simulink model "foc"  (R2023a)
settings: Solver=VariableStepAuto  StartTime=0.0  StopTime=20  FixedStep=1e-4  MaxStep=1e-4  RelTol=1e-3
values from neighbouring files (symbols this model uses):
  A = exp(F*Ts)    [data.m]
  V = 12    [data.m]
libraries: spsMosfetLib x6, spsPermanentMagnetSynchronousMachineLib x1, spsCurrentMeasurementLib x1, spsDCVoltageSourceLib x1, spsGroundLib x1, slpidlib x1, simulink x1, mcbsensorlessestimatorlib x1, sps_lib x1
settings Model: Creator=Daniil  LastModifiedBy=Daniil

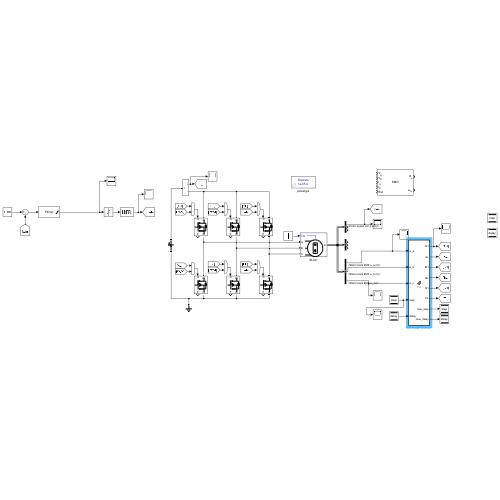
[thumbnail: Simulink's stored preview of the top-level diagram]
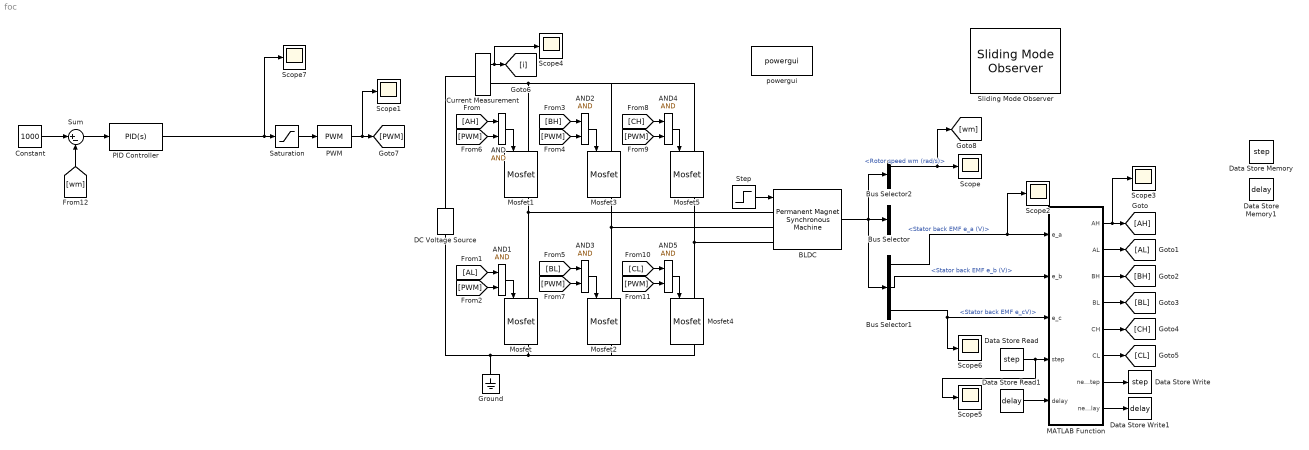
== system foc ==
  AND{,1..5} (6 alike) : Logic  IconShape=distinctive  AllPortsSameDT=off  OutDataTypeStr=boolean
  BLDC : spsPermanentMagnetSynchronousMachineLib/Permanent Magnet Synchronous Machine  NbPhases=3  FluxDistribution=Trapezoidal  RotorType=Round  MechanicalLoad=Torque Tm  PresetModel=No  ShowDetailedParameters=on  MeasurementBus=off  Resistance=0.18  Inductance=0.000835  dqInductances=[8.5e-3,8.5e-3]  La=0.000835  MachineConstant=Flux linkage established by magnets (V.s)  Flux=0.00108515  VoltageCst=0.90909  TorqueCst=0.0086812  Flat=120  Mechanical=[0.0621417 0.000303448 4]  PolePairs=4  InitialConditions=[10,0, 0,0]  InitialConditions5ph=[0 0 0 0 0 0]  RefAngle=90 degrees behind phase A axis (modified Park)  IterativeDiscreteModel=Trapezoidal non iterative  TsBlock=-1  TsPowergui=0
  Bus Selector : BusSelector  OutputSignals=Stator current is_a (A),Stator current is_b (A),Stator current is_c (A)
  Bus Selector1 : BusSelector  OutputSignals=Stator back EMF e_a (V),Stator back EMF e_b (V),Stator back EMF e_cV)
  Bus Selector2 : BusSelector  OutputSignals=Rotor speed wm (rad/s),Rotor angle thetam (rad),Electromagnetic torque Te (N*m)
  Constant : Constant  Value=1000
  Current Measurement : spsCurrentMeasurementLib/Current Measurement  PhasorSimulation=off  OutputType=Complex  PSBequivalent=0
  DC Voltage Source : spsDCVoltageSourceLib/DC Voltage Source  Amplitude=12  Measurements=None
  Data Store Memory : DataStoreMemory  DataStoreName=step  WriteAfterWriteMsg=warning  ShowAdditionalParam=off
  Data Store Memory1 : DataStoreMemory  DataStoreName=delay  WriteAfterWriteMsg=warning  ShowAdditionalParam=off
  Data Store Read : DataStoreRead  DataStoreName=step  IndexOptions=Index vector (dialog)  Indices=1  OutputSizes=1
  Data Store Read1 : DataStoreRead  DataStoreName=delay  IndexOptions=Index vector (dialog)  Indices=1  OutputSizes=1
  Data Store Write : DataStoreWrite  DataStoreName=step  IndexOptions=Index vector (dialog)  Indices=1  OutputSizes=1
  Data Store Write1 : DataStoreWrite  DataStoreName=delay  IndexOptions=Index vector (dialog)  Indices=1  OutputSizes=1
  Ground : spsGroundLib/Ground  LConnTagsString=a
  MATLAB Function : MATLAB Function  TreatAsAtomicUnit=on
  Mosfet{,1..5} (6 alike) : spsMosfetLib/Mosfet  Ron=0.1  Lon=0  Rd=0.01  Vfd=0  IC=0  Rs=1e5  Cs=inf  Measurements=on
  PID Controller : slpidlib/PID Controller  Controller=PID  Form=Parallel  TimeDomain=Continuous-time  UseExternalTs=off  SampleTime=-1  IntegratorMethod=Forward Euler  FilterMethod=Forward Euler  ControllerParametersSource=internal  P=10000  I=10  UseKiTs=off  D=0  N=100  UseFilter=on  TunerSelectOption=Transfer Function Based (PID Tuner App)  InitialConditionSource=internal  InitialConditionForIntegrator=0  InitialConditionForFilter=0  DifferentiatorICPrevScaledInput=0  ExternalReset=none  TrackingMode=off  Kt=1  LimitOutput=on  SatLimitsSource=internal  UpperSaturationLimit=1  LowerSaturationLimit=0  LinearizeAsGain=on  AntiWindupMode=none  Kb=1  LimitIntegrator=off  UpperIntegratorSaturationLimit=inf  LowerIntegratorSaturationLimit=-inf  POutMin=[]  POutMax=[]  IOutMin=[]  IOutMax=[]  DOutMin=[]  DOutMax=[]  NOutMin=[]  NOutMax=[]  SumOutMin=[]  SumOutMax=[]  SaturationOutMin=[]  SaturationOutMax=[]  PParamMin=[]  PParamMax=[]  IParamMin=[]  IParamMax=[]  DParamMin=[]  DParamMax=[]  NParamMin=[]  NParamMax=[]  KbParamMin=[]  KbParamMax=[]  KtParamMin=[]  KtParamMax=[]  KbOutMin=[]  KbOutMax=[]  KtOutMin=[]  KtOutMax=[]  IntegratorOutMin=[]  IntegratorOutMax=[]  FilterOutMin=[]  FilterOutMax=[]  SumI1OutMin=[]  SumI1OutMax=[]  SumI2OutMin=[]  SumI2OutMax=[]  SumI3OutMin=[]  SumI3OutMax=[]  SumI4OutMin=[]  SumI4OutMax=[]  SumDOutMin=[]  SumDOutMax=[]  DifferentiatorOutMin=[]  DifferentiatorOutMax=[]  FilterDiffOutCoefMin=[]  FilterDiffOutCoefMax=[]  ReciprocalOutMin=[]  ReciprocalOutMax=[]  SumDenOutMin=[]  SumDenOutMax=[]  SumNumOutMin=[]  SumNumOutMax=[]  DivideOutMin=[]  DivideOutMax=[]  UdiffTsProdOutMin=[]  UdiffTsProdOutMax=[]  NTsProdOutMin=[]  NTsProdOutMax=[]  UintegralTsProdOutMin=[]  UintegralTsProdOutMax=[]  UngainTsProdOutMin=[]  UngainTsProdOutMax=[]  ClampingZeroOutDataTypeStr=Inherit: Inherit via back propagation  ClampingZeroOutMin=[]  ClampingZeroOutMax=[]  FilterDenConstantOutDataTypeStr=Inherit: Inherit via back propagation  FilterDenConstantOutMin=[]  FilterDenConstantOutMax=[]  PCopyOutDataTypeStr=Inherit: Inherit via back propagation  PCopyOutMin=[]  PCopyOutMax=[]  NCopyOutDataTypeStr=Inherit: Inherit via back propagation  NCopyOutMin=[]  NCopyOutMax=[]  IntegratorContinuousStateAttributes=''  IntegratorStateMustResolveToSignalObject=off  IntegratorRTWStateStorageClass=Auto  FilterContinuousStateAttributes=''  FilterStateMustResolveToSignalObject=off  FilterRTWStateStorageClass=Auto  ParallelPVariant=InternalParameters  IdealPVariant=Disabled  IVariant=InternalParameters  DVariant=InternalParameters  IntegratorVariant=Continuous  SatVariant=Enabled  AWVariant=Passthrough  PCopyVariant=Disabled  TRVariant=Disabled  FdbkBlocksVariant=Forward  IdealPFdbkVariant=Disabled  SatFdbkVariant=Disabled  DerivativeFilterVariant=ContFilter  NVariant=InternalParameters  NCopyVariant=Disabled  FilterICVariant=InternalICsFilter  IntegratorICVariant=InternalICs  ExternalResetVariant=Disabled  TRSumVariant=Passthrough  SumFdbkVariant=Disabled  SumVariant=Sum_PID  TsampFilterVariant=InternalTs  TsampNgainVariant=Passthrough  TsampIntegralVariant=Disabled_SignalSpec  ExternalSaturationOutDataTypeStr=Inherit: Same as second input
  PWM : simulink/Discontinuities/PWM  DisableCoverage=on  Period=0.001  InitialDelay=0  DisallowZeroDutyCycle=off  RunAtFixedTimeIntervals=off  SampleTime=0.1
  Saturation : Saturate  UpperLimit=1  LowerLimit=0
  Scope{,1..7} (8 alike) : Scope
  Sliding Mode Observer : mcbsensorlessestimatorlib/Sliding Mode Observer  InputUnit=SI unit  BlkSampleTime=50e-6  StatorResistance=0.36  StatorInductance=0.2e-3  MaxApplicationSpeed=6000  PolePairs=4  MaxStatorVoltage=13.8564  MaxStatorCurrent=21.4286  DisturbanceObserverGain=0.9  CurrentObserverGain=0.50881  CutoffFreq=1200  PositionUnit=Degrees  PositionDataType=single  SpeedUnit=Degrees/sec  PerUnitSpeed=6000  SpeedDataType=single
      settings: LibrarySourceBlock=mcblib/Sensorless Estimators/Sliding Mode Observer
  Step : Step  After=0  SampleTime=0
  Sum : Sum  Inputs=|+-
  powergui : sps_lib/powergui  Priority=1  SimulationMode=Discrete  SampleTime=1e-5  frequency=60  Iterations=50  frequencyindice=0  Pbase=100e6  ErrMax=1e-4  UnitsV=kV  UnitsW=MW  buscounter=0  FunctionMessages=off  echomessages=off  EnableUseOfTLC=off  CurrentSourceSwitches=off  DisableSnubberDevices=off  DisableRonSwitches=off  DisableVfSwitches=off  DisplayEquations=off  AutomaticDiscreteSolvers=off  SolverType=Tustin/Backward Euler (TBE)  Interpol=off  ExternalGateDelay=off  methode=off  Ts=100  x0status=blocks  SPID=on  SwTol=0  HookPort=off  NonlinearTolerance=1e-4  nMaxIteration=100  ContinueOnMaxIteration=off  RestoreLinks=warning  ResistiveCurrentMeasurement=off  Frange=[0:2:500]  Ylog=off  Xlog=on  ShowGrid=off  save=off  variable=ZData  structure=0  ZoomFFT=off  StartTime=0.0  cycles=1  DisplayStyle=1  fundamental=60  FreqAxis=off  MaxFrequency=1000  frequencyindicesteady=1  RmsSteady=1  display=off
  wires:
  Step/1 -> BLDC/1
  BLDC/1 -> Bus Selector2/1, Bus Selector1/1, Bus Selector/1
  Bus Selector1/2 -> MATLAB Function/2(e_b)  "<Stator back EMF e_b (V)>"
  Bus Selector1/3 -> Scope6/1, MATLAB Function/3(e_c)  "<Stator back EMF e_cV)>"
  Bus Selector1/1 -> Scope2/1, MATLAB Function/1(e_a)  "<Stator back EMF e_a (V)>"
  MATLAB Function/1(AH) -> Scope3/1, [AH]
  MATLAB Function/2(AL) -> [AL]
  MATLAB Function/3(BH) -> [BH]
  MATLAB Function/4(BL) -> [BL]
  MATLAB Function/5(CH) -> [CH]
  MATLAB Function/6(CL) -> [CL]
  Bus Selector2/1 -> [wm], Scope/1  "<Rotor speed wm (rad/s)>"
  Data Store Read/1 -> Scope5/1, MATLAB Function/4(step)
  Saturation/1 -> PWM/1
  Current Measurement/1 -> Scope4/1, [i]
  AND/1 -> Mosfet1/1
  [PWM] -> AND/2
  [AH] -> AND/1
  AND1/1 -> Mosfet/1
  [PWM] -> AND1/2
  [AL] -> AND1/1
  AND2/1 -> Mosfet3/1
  [PWM] -> AND2/2
  [BH] -> AND2/1
  AND3/1 -> Mosfet2/1
  [BL] -> AND3/1
  [PWM] -> AND3/2
  AND4/1 -> Mosfet5/1
  [CH] -> AND4/1
  [PWM] -> AND4/2
  PWM/1 -> Scope1/1, [PWM]
  AND5/1 -> Mosfet4/1
  [PWM] -> AND5/2
  [CL] -> AND5/1
  [wm] -> Sum/2
  Sum/1 -> PID Controller/1
  Constant/1 -> Sum/1
  MATLAB Function/7(new_step) -> Data Store Write/1
  Data Store Read1/1 -> MATLAB Function/5(delay)
  MATLAB Function/8(new_delay) -> Data Store Write1/1
  PID Controller/1 -> Scope7/1, Saturation/1
  connections:
  Mosfet1/RConn1 -- BLDC/LConn1 -- Mosfet/LConn1
  DC Voltage Source/RConn1 -- Current Measurement/LConn1
  DC Voltage Source/LConn1 -- Mosfet4/RConn1 -- Mosfet2/RConn1 -- Mosfet/RConn1 -- Ground/LConn1
  Mosfet1/LConn1 -- Mosfet3/LConn1 -- Mosfet5/LConn1 -- Current Measurement/RConn1
  Mosfet3/RConn1 -- Mosfet2/LConn1 -- BLDC/LConn2
  Mosfet5/RConn1 -- Mosfet4/LConn1 -- BLDC/LConn3

== matlab function foc/MATLAB Function ==
  data: e_a input; AH output; e_b input; e_c input; AL output; BH output; BL output; CH output; CL output; step input; new_step output; delay input; new_delay output
function [AH, AL, BH, BL, CH, CL, new_step, new_delay] = fcn(e_a, e_b, e_c, step, delay)

delta = 1e-5;
delay_max = 50;

cur_bemf_check = 10000;

switch step
    case 0
        AH = 1;
        AL = 0;
        BH = 0;
        BL = 1;
        CH = 0;
        CL = 0;
        cur_bemf_check = e_c;
    case 1
        AH = 1;
        AL = 0;
        BH = 0;
        BL = 0;
        CH = 0;
        CL = 1;
        cur_bemf_check = e_b;
    case 2
        AH = 0;
        AL = 0;
        BH = 1;
        BL = 0;
        CH = 0;
        CL = 1;
        cur_bemf_check = e_a;
    case 3
        AH = 0;
        AL = 1;
        BH = 1;
        BL = 0;
        CH = 0;
        CL = 0;
        cur_bemf_check = e_c;
    case 4
        AH = 0;
        AL = 1;
        BH = 0;
        BL = 0;
        CH = 1;
        CL = 0;
        cur_bemf_check = e_b;
    case 5
        AH = 0;
        AL = 0;
        BH = 0;
        BL = 1;
        CH = 1;
        CL = 0;
        cur_bemf_check = e_a;
    otherwise
        AH = 1;
        AL = 0;
        BH = 0;
        BL = 1;
        CH = 0;
        CL = 0;
end

if abs(cur_bemf_check) < delta && delay >= delay_max
    new_delay = 0;
    new_step = step + 1;
    if new_step > 5
        new_step = 0;
    end
else
    new_delay = delay + 1;
    new_step = step;
end
